simulink model "MRAR"  (R2023b)
settings: Solver=ode45  StartTime=0.0  StopTime=20  RelTol=1e-3
values from neighbouring files (symbols this model uses):
  b1 = 1000    [Condiciones.mat]    (also in MRAM.m; ODE_MRAR2.m)
  k1 = 16182    [Condiciones.mat]    (also in MRAM.m; ODE_MRAR2.m)
  k2 = 19000    [Condiciones.mat]    (also in MRAM.m; ODE_MRAR2.m)
  m1 = 290    [Condiciones.mat]    (also in MRAM.m; ODE_MRAR2.m)
  m2 = 59    [Condiciones.mat]    (also in MRAM.m; ODE_MRAR2.m)
settings Model: Creator=andre  LastModifiedBy=andre

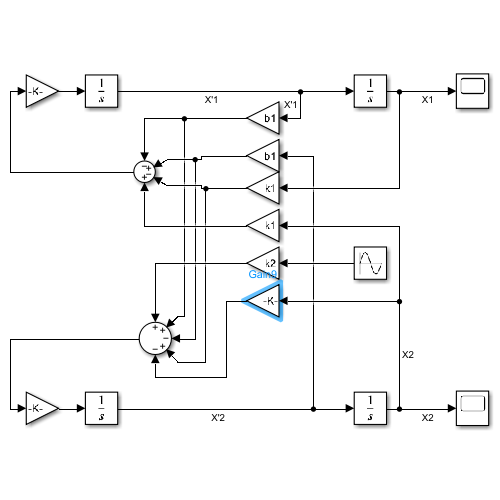
[thumbnail: Simulink's stored preview of the top-level diagram]
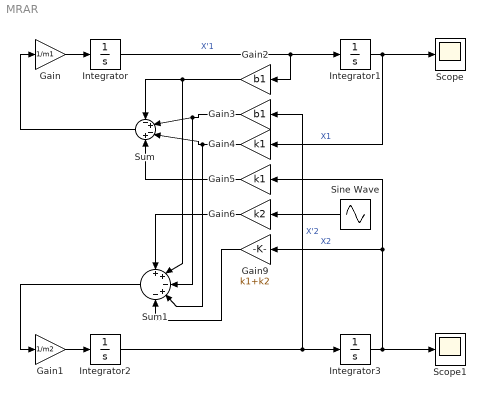
== system MRAR ==
  Gain : Gain  Gain=1/m1
  Gain1 : Gain  Gain=1/m2
  Gain2 : Gain  Gain=b1
  Gain3 : Gain  Gain=b1
  Gain4 : Gain  Gain=k1
  Gain5 : Gain  Gain=k1
  Gain6 : Gain  Gain=k2
  Gain9 : Gain  Gain=k1+k2
  Integrator{,1..3} (4 alike) : Integrator
  Scope : Scope
  Scope1 : Scope
  Sine Wave : Sin  Amplitude=0.05  Frequency=0.5*pi  SampleTime=0
  Sum : Sum  Inputs=-+-+
  Sum1 : Sum  Inputs=++-+-
  wires:
  Integrator/1 -> Integrator1/1, Gain2/1  "X'1"
  Integrator1/1 -> Gain4/1, Scope/1  "X1"
  Integrator3/1 -> Scope1/1, Gain9/1, Gain5/1  "X2"
  Integrator2/1 -> Gain3/1, Integrator3/1  "X'2"
  Gain/1 -> Integrator/1
  Sum/1 -> Gain/1
  Gain1/1 -> Integrator2/1
  Sum1/1 -> Gain1/1
  Gain2/1 -> Sum1/2, Sum/1
  Gain3/1 -> Sum1/3, Sum/2
  Gain4/1 -> Sum1/4, Sum/3
  Gain5/1 -> Sum/4
  Gain6/1 -> Sum1/1
  Sine Wave/1 -> Gain6/1
  Gain9/1 -> Sum1/5
